simulink model "UNCONTROLLED_3PH_RECTIFIER"  (R2025a)
settings: Solver=VariableStepAuto  StartTime=0.0  StopTime=0.1  RelTol=1e-3
libraries: spsDiodeLib x6, spsACVoltageSourceLib x3, spsMultimeterLib x2, spsSeriesRLCBranchLib x1, sps_lib x1
settings Model: Creator=samar  LastModifiedBy=samar

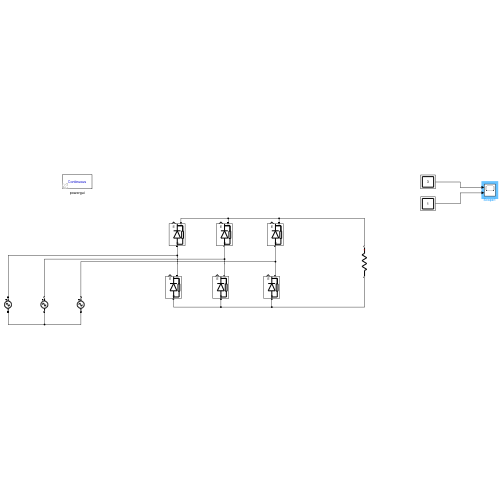
[thumbnail: Simulink's stored preview of the top-level diagram]
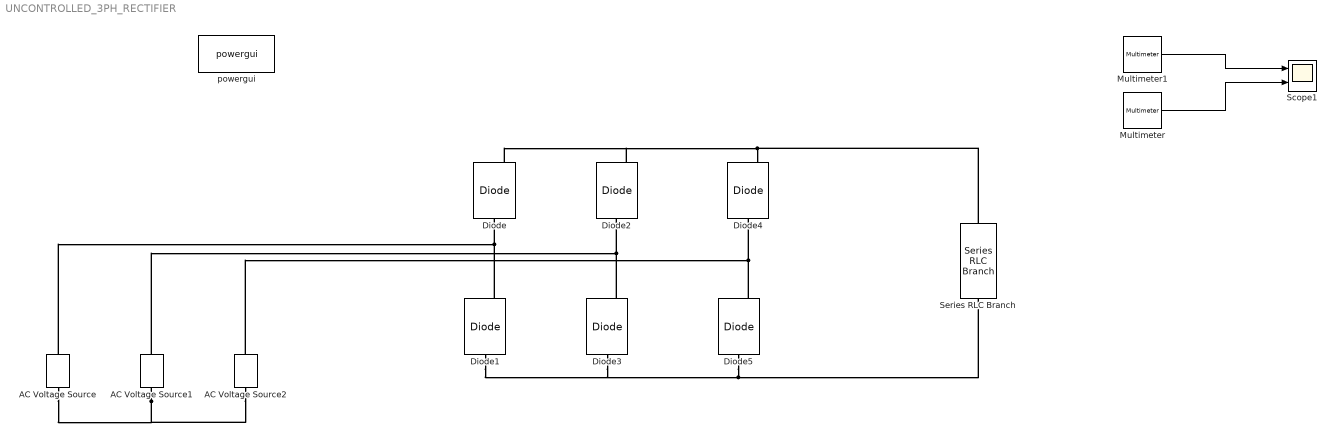
== system UNCONTROLLED_3PH_RECTIFIER ==
  AC Voltage Source : spsACVoltageSourceLib/AC Voltage Source  Amplitude=100  Phase=0  Frequency=50  SampleTime=0  Measurements=Voltage  BusType=swing  Pref=10e3  Qref=0  Qmin=-inf  Qmax=+inf
  AC Voltage Source1 : spsACVoltageSourceLib/AC Voltage Source  Amplitude=100  Phase=-120  Frequency=50  SampleTime=0  Measurements=Voltage  BusType=swing  Pref=10e3  Qref=0  Qmin=-inf  Qmax=+inf
  AC Voltage Source2 : spsACVoltageSourceLib/AC Voltage Source  Amplitude=100  Phase=-240  Frequency=50  SampleTime=0  Measurements=Voltage  BusType=swing  Pref=10e3  Qref=0  Qmin=-inf  Qmax=+inf
  Diode{,1..5} (6 alike) : spsDiodeLib/Diode  Ron=0.001  Lon=0  Vf=0.8  IC=0  UseSnubber=0  Rs=500  Cs=250e-9  Measurements=on
  Multimeter : spsMultimeterLib/Multimeter  L=4  sel=1  yselected={}  Gain=1  OutputType=Complex  PlotAtSimulationStop=off  PhasorSimulation=off
  Multimeter1 : spsMultimeterLib/Multimeter  L=4  sel=[2 3 4]  yselected={}  Gain=[1 1 1]  OutputType=Complex  PlotAtSimulationStop=off  PhasorSimulation=off
  Scope1 : Scope  NumInputPorts=2
      settings: ActiveDisplayYMinimum=-124.99681861392463  ActiveDisplayYMaximum=124.97281119951293
  Series RLC Branch : spsSeriesRLCBranchLib/Series RLC Branch  LConnTagsString=__new0  RConnTagsString=__new0  BranchType=R  Resistance=100  Inductance=1e-3  SetiL0=off  InitialCurrent=0  Capacitance=1e-6  Setx0=off  InitialVoltage=0  Measurements=Branch voltage
  powergui : sps_lib/powergui  Priority=1  SimulationMode=Continuous  SampleTime=50e-6  frequency=60  Iterations=50  frequencyindice=50  Pbase=100e6  ErrMax=1e-4  UnitsV=kV  UnitsW=MW  buscounter=0  FunctionMessages=off  echomessages=off  EnableUseOfTLC=off  CurrentSourceSwitches=off  DisableSnubberDevices=off  DisableRonSwitches=off  DisableVfSwitches=off  DisplayEquations=off  AutomaticDiscreteSolvers=off  SolverType=Tustin/Backward Euler (TBE)  Interpol=off  ExternalGateDelay=off  methode=off  Ts=100  x0status=blocks  SPID=on  SwTol=0  HookPort=off  NonlinearTolerance=1e-4  nMaxIteration=100  ContinueOnMaxIteration=off  RestoreLinks=warning  ResistiveCurrentMeasurement=off  Frange=[0:2:500]  Ylog=off  Xlog=on  ShowGrid=off  save=off  variable=ZData  structure=0  ZoomFFT=off  StartTime=0.0  cycles=1  DisplayStyle=1  fundamental=60  FreqAxis=off  MaxFrequency=1000  frequencyindicesteady=1  RmsSteady=1  display=off
  wires:
  Multimeter/1 -> Scope1/2
  Multimeter1/1 -> Scope1/1
  connections:
  AC Voltage Source1/LConn1 -- AC Voltage Source/LConn1 -- AC Voltage Source2/LConn1
  Diode1/RConn1 -- AC Voltage Source/RConn1 -- Diode/LConn1
  Diode5/LConn1 -- Diode3/LConn1 -- Diode1/LConn1 -- Series RLC Branch/RConn1
  Series RLC Branch/LConn1 -- Diode/RConn1 -- Diode2/RConn1 -- Diode4/RConn1
  Diode3/RConn1 -- AC Voltage Source1/RConn1 -- Diode2/LConn1
  Diode5/RConn1 -- AC Voltage Source2/RConn1 -- Diode4/LConn1
